simulink model "METI_Thermal_ver01_Jmaab_2018b_Intg"  (R2018b)
settings: Solver=ode8  StartTime=0  StopTime=end_time  FixedStep=sampling_time  RelTol=1e-3
PreLoadFcn:
  | %init_setting;
values from neighbouring files (symbols this model uses):
  degC2K = 273.15    [METI_TRAMI_Thermal_ver01_Jmaab_PreLoad.m]    (also in init_setting_METI.m)
  K2degC = -273.15    [METI_TRAMI_Thermal_ver01_Jmaab_PreLoad.m]    (also in init_setting_METI.m)
  sampling_time = 0.0025    [METI_TRAMI_Thermal_ver01_Jmaab_PreLoad.m]
undefined symbols (not defined in the file or in its folder): ACC_D_Gain, ACC_I_Gain, ACC_P_Gain, ALT_CNT_ALT_OFF_RPM_HYS_rpm, ALT_CNT_ALT_ON_RPM_HYS_rpm, ALT_CNT_Alter_V_BASE_V, ALT_CNT_Alter_V_Kaisei_V, ALT_CNT_flag_disable_kaisei, ALT_CNT_V_Battely_Kudo_V, ALT_PNT_ALT_GDCurrent_A, ALT_PNT_ALT_GDVolt_V, ALT_PNT_Alter_limit_Current_V_table, ALT_PNT_Alter_limit_Current_V_table_x_rpm, ALT_PNT_Alter_trq_Nm_map, ALT_PNT_Alter_trq_Nm_map_x_rpm, ALT_PNT_Alter_trq_Nm_map_y_Current_A, ALT_PNT_Alter_trq_Nm_map_z_Volt_tgt_V, ALT_PNT_eta_pulley_alt, ALT_PNT_Gain_Alt_v_del, ALT_PNT_ratio_pulley_alt, ALT_PNT_Tau_Alternator_V_tgt_s, ALT_PNT_trq_alter_output_LL_Nm, BK_PNT_Pow_UL, BK_PNT_Tau_brake, Brk_LL, Brk_PGain, Brk_UL, BT_PNT_Lo_Capa_lo_batt_F, BT_PNT_Lo_ocv_SOC_lo_batt_OCV_V_table, BT_PNT_Lo_ocv_SOC_lo_batt_OCV_V_table_x_SOC, BT_PNT_Lo_R_lo_batt_ohm, BT_PNT_Lo_SOC_MAX_lo_batt, BT_PNT_Lo_SOC_MIN_lo_batt, BT_PNT_Lo_SOC_START_lo_batt, BT_PNT_Lo_V_start_ocv, DF_PNT_DF_gear, DF_PNT_DFBlock2DFAir_Heat_Resi_KpW, DF_PNT_DFBlock_Heat_Capa_JpK, DF_PNT_DFBlock_Temp_ini_degC, DF_PNT_DFOil2DFBlock_Heat_Resi_KpW, DF_PNT_DFOil_Heat_Capa_JpK, DF_PNT_DFOil_Temp_ini_degC, DF_PNT_Driveshaft_damper, DF_PNT_Driveshaft_delta_radps_LL, DF_PNT_Driveshaft_delta_radps_UL, DF_PNT_Driveshaft_spring, DF_PNT_eta_DF, DF_PNT_Outtemp_degC, DF_PNT_TMBlock2DFBlock_Heat_Resi_KpW, Driver_Brake_Const1, Driver_Brake_Const3, Driver_Brake_Switch_Const2, Driver_Brk_sh, drivmode_ACC, drivmode_CONST, drivmode_GensokuKaisei, drivmode_GensokuRikko, drivmode_STOP, EL_PNT_R_bodyelec_lo_ohm, ENG_CNT_acc_idlestop ... (+137)
libraries: METI_Lib_vehicle_model x31, simulink x7, AZAPA_Lib_vehicle_model x1
(part 2 of 4)

== system METI_Thermal_ver01_Jmaab_2018b_Intg/Vehicle/CNT/ENG_CNT ==
  Driver_Input : Inport
  sensor_ENG_PNT : Inport  Port=2
  Bus Creator : BusCreator  Inputs=5
  Bus Creator1 : BusCreator  Inputs=10
  Bus Selector1 : BusSelector  OutputSignals=v_VL_PNT_kmph,flag_Lockup
  Bus Selector13 : BusSelector  OutputSignals=n_eng_rpm,fuel_consumption,T_ENGTH_PNT_Coolant_degC
  Bus Selector14 : BusSelector  OutputSignals=open_accel_per,open_brake_per
  ENG_Cntrl : Subsystem
  ENG_CNT_out : Outport
  tag scope: ENG_CNT_CAN_Tx=scoped
  wires:
  Bus Creator/1 -> [ENG_CNT_CAN_Tx]  "ENG_CNT_CAN_Tx"
  ENG_Cntrl/1(open_throttle_per) -> Bus Creator/1, Bus Creator1/1
  ENG_Cntrl/2(flag_IdleStop) -> Bus Creator/2, Bus Creator1/2
  ENG_Cntrl/3(flag_fuelcut) -> Bus Creator/3, Bus Creator1/3
  ENG_Cntrl/4(fuel_ratio) -> Bus Creator1/4
  ENG_Cntrl/5(timing_ignition) -> Bus Creator1/5
  ENG_Cntrl/6(n_eng_rpm) -> Bus Creator/4, Bus Creator1/6
  ENG_Cntrl/7(flag_ON_Starter) -> Bus Creator1/7
  Bus Creator1/1 -> ENG_CNT_out/1  "ENG_CNT_out"
  sensor_ENG_PNT/1 -> Bus Selector13/1
  Bus Selector13/1 -> ENG_Cntrl/3(sens_ENG_PNT)  "<n_eng_rpm>"
  Driver_Input/1 -> Bus Selector14/1
  Bus Selector14/1 -> ENG_Cntrl/1(open_accel_per)  "<open_accel_per>"
  Bus Selector14/2 -> ENG_Cntrl/2(open_brake_per)  "<open_brake_per>"
  [ENG_CNT_CAN_Rx] -> Bus Selector1/1
  Bus Selector1/2 -> ENG_Cntrl/7(flag_Lockup)  "<flag_Lockup>"
  ENG_Cntrl/8(K_Fuel) -> Bus Creator1/8
  ENG_Cntrl/9(V_ENG_CNT_WP_V) -> Bus Creator1/9
  ENG_Cntrl/10(V_ENG_CNT_RDFan_V) -> Bus Creator1/10
  Bus Selector13/2 -> ENG_Cntrl/4(fuel_consumption)  "<fuel_consumption>"
  Bus Selector13/3 -> Bus Creator/5, ENG_Cntrl/5(T_ENGTH_PNT_Coolant_degC)  "<T_ENGTH_PNT_Coolant_degC>"
  Bus Selector1/1 -> ENG_Cntrl/6(v_VL_PNT_kmph)  "<v_VL_PNT_kmph>"

== system METI_Thermal_ver01_Jmaab_2018b_Intg/Vehicle/CNT/TM_CNT ==
  sensor_TM_PNT : Inport
  Rate Transition : RateTransition  Deterministic=off
      settings: AttributesFormatString=|
      | <Integrity = %<Integrity>>
      | <Deterministic = %<Deterministic>>
  Rate Transition1 : RateTransition  Deterministic=off
      settings: AttributesFormatString=|
      | <Integrity = %<Integrity>>
      | <Deterministic = %<Deterministic>>
  Rate Transition2 : RateTransition  Deterministic=off
      settings: AttributesFormatString=|
      | <Integrity = %<Integrity>>
      | <Deterministic = %<Deterministic>>
  TM_CNT : Subsystem  TreatAsAtomicUnit=on
      settings: AttributesFormatString="<AtomicUnit =  %<TreatAsAtomicUnit>>"
  TM_CNT_out : Outport
  tag scope: TM_CNT_CAN_Tx=scoped, TM_CNT_Info=global
  wires:
  sensor_TM_PNT/1 -> Rate Transition/1
  [TM_CNT_CAN_Rx] -> Rate Transition1/1
  TM_CNT/1(TM_CNT_out) -> Rate Transition2/1
  TM_CNT/2(TM_CNT_CAN_Tx) -> [TM_CNT_CAN_Tx]
  TM_CNT/3(TM_CNT_Info) -> [TM_CNT_Info]
  Rate Transition/1 -> TM_CNT/1(sensor_TM_PNT_BUS)
  Rate Transition1/1 -> TM_CNT/2(TM_CNT_CAN_Rx)
  Rate Transition2/1 -> TM_CNT_out/1  "TM_CNT_out"

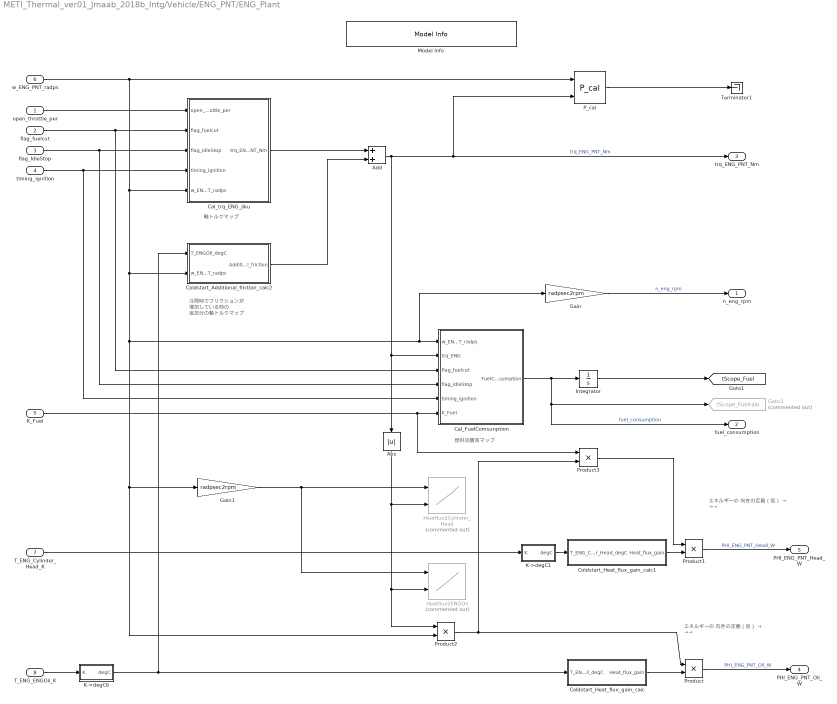
== system METI_Thermal_ver01_Jmaab_2018b_Intg/Vehicle/ENG_PNT/ENG_Plant ==
  note: 軸トルクマップ
  note: 燃料消費率マップ
  note: 冷間時でフリクションが
      | 増加している時の
      | 追加分の軸トルクマップ
  note: エネルギーの
      | 向きの定義（仮）
      | → →→
  note: エネルギーの
      | 向きの定義（仮）
      | → →→
  open_throttle_per : Inport
  flag_fuelcut : Inport  Port=2
  flag_IdleStop : Inport  Port=3
  timing_ignition : Inport  Port=4
  K_Fuel : Inport  Port=5
  w_ENG_PNT_radps : Inport  Port=6
  T_ENG_Cylinder_Head_K : Inport  Port=7
  T_ENG_ENGOil_K : Inport  Port=8
  Abs : Abs
  Add : Sum
  Cal_FuelComsunption : Subsystem
  Cal_trq_ENG_jiku : Subsystem
  Coldstart_Additional_friction_calc2 : Subsystem
  Coldstart_Heat_flux_gain_calc : Subsystem
  Coldstart_Heat_flux_gain_calc1 : Subsystem
  Gain : Gain  Gain=radpsec2rpm
  Gain1 : Gain  Gain=radpsec2rpm
  Goto3 : Goto  Commented=on  GotoTag=tScope_Fuelraio  TagVisibility=global
  Heatflux2Cylinder_Head : Lookup_n-D  Commented=on  BreakpointsForDimension1=ENG_PNT_Heatflux2Cylinder_Head_W_x_rpm  BreakpointsForDimension2=ENG_PNT_Heatflux2Cylinder_Head_W_y_trq  Table=ENG_PNT_Heatflux2Cylinder_Head_W  InternalRulePriority=Speed  RndMeth=Simplest  InputSameDT=on
  Heatflux2ENGOil : Lookup_n-D  Commented=on  BreakpointsForDimension1=ENG_PNT_Heatflux2ENGOil_W_x_rpm  BreakpointsForDimension2=ENG_PNT_Heatflux2ENGOil_W_y_trq  Table=ENG_PNT_Heatflux2ENGOil_W  InternalRulePriority=Speed  RndMeth=Simplest  InputSameDT=on
  Integrator : Integrator
  K->degC1 : Subsystem
  K->degC6 : Subsystem
  Model Info : simulink/Model-Wide Utilities/Model Info  Frame=on  DisplayStringWithTags=【注記】 ・エンジンモデルはトルク出力動作させる側が正  HorizontalTextAlignment=Left  LeftAlignmentValue=0.02
  P_cal : METI_Lib_vehicle_model/P_cal  Type_energy=回転運動  Type_output_energy=出力  Power_name=Po_  t_Workspace_Name=ENG_PNT_MECK  P_VariableName=Po_ENG_PNT_MECK  Across_VariableName=w_ENG_PNT_MECK  Throgh_VariableName=tq_ENG_PNT_MECK
  Product{,1..3} (4 alike) : Product
  Terminator1 : Terminator
  n_eng_rpm : Outport
  fuel_consumption : Outport  Port=2
  trq_ENG_PNT_Nm : Outport  Port=3
  PHI_ENG_PNT_Oil_W : Outport  Port=4
  PHI_ENG_PNT_Head_W : Outport  Port=5
  tag scope: tScope_Fuel=global
  wires:
  Cal_FuelComsunption/1(FuelConsumption) -> fuel_consumption/1, Goto3/1, Integrator/1  "fuel_consumption"
  Integrator/1 -> [tScope_Fuel]
  w_ENG_PNT_radps/1 -> P_cal/1, Coldstart_Additional_friction_calc2/2(w_ENG_PNT_radps), Gain1/1, Product2/2, Gain/1, Cal_FuelComsunption/1(w_ENG_PNT_radps), Cal_trq_ENG_jiku/5(w_ENG_PNT_radps)
  P_cal/1 -> Terminator1/1
  flag_fuelcut/1 -> Cal_trq_ENG_jiku/2(flag_fuelcut), Cal_FuelComsunption/3(flag_fuelcut)
  flag_IdleStop/1 -> Cal_FuelComsunption/4(flag_IdleStop), Cal_trq_ENG_jiku/3(flag_IdleStop)
  open_throttle_per/1 -> Cal_trq_ENG_jiku/1(open_throttle_per)
  Cal_trq_ENG_jiku/1(trq_ENG_PNT_Nm) -> Add/1
  timing_ignition/1 -> Cal_FuelComsunption/5(timing_ignition), Cal_trq_ENG_jiku/4(timing_ignition)
  Gain/1 -> n_eng_rpm/1  "n_eng_rpm"
  K->degC6/1(degC) -> Coldstart_Heat_flux_gain_calc/1(T_ENGOil_degC), Coldstart_Additional_friction_calc2/1(T_ENGOil_degC)
  T_ENG_Cylinder_Head_K/1 -> K->degC1/1(K)
  Product1/1 -> PHI_ENG_PNT_Head_W/1  "PHI_ENG_PNT_Head_W"
  Product/1 -> PHI_ENG_PNT_Oil_W/1  "PHI_ENG_PNT_Oil_W"
  Gain1/1 -> Heatflux2ENGOil/1, Heatflux2Cylinder_Head/1
  Coldstart_Heat_flux_gain_calc/1(Heat_flux_gain) -> Product/2
  Product2/1 -> Product/1, Product3/2
  Coldstart_Heat_flux_gain_calc1/1(Heat_flux_gain) -> Product1/2
  Coldstart_Additional_friction_calc2/1(Additional_friction) -> Add/2
  Add/1 -> trq_ENG_PNT_Nm/1, P_cal/2, Cal_FuelComsunption/2(trq_ENG), Abs/1  "trq_ENG_PNT_Nm"
  K_Fuel/1 -> Product3/1, Cal_FuelComsunption/6(K_Fuel)
  Abs/1 -> Product2/1, Heatflux2ENGOil/2, Heatflux2Cylinder_Head/2
  Product3/1 -> Product1/1
  T_ENG_ENGOil_K/1 -> K->degC6/1(K)
  K->degC1/1(degC) -> Coldstart_Heat_flux_gain_calc1/1(T_ENG_Cylinder_Head_degC)

== system METI_Thermal_ver01_Jmaab_2018b_Intg/Vehicle/ENG_PNT/K->degC ==
  K : Inport
  Constant2 : Constant  Value=K2degC
  Sum : Sum  Inputs=++|
  degC : Outport
  wires:
  K/1 -> Sum/2
  Constant2/1 -> Sum/1
  Sum/1 -> degC/1

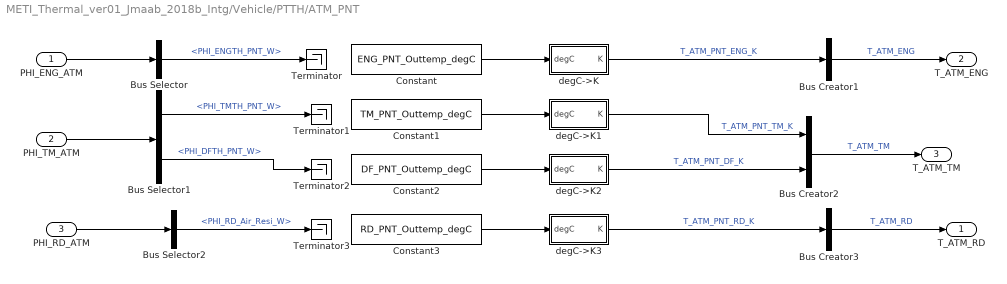
== system METI_Thermal_ver01_Jmaab_2018b_Intg/Vehicle/PTTH/ATM_PNT ==
  PHI_ENG_ATM : Inport
  PHI_TM_ATM : Inport  Port=2
  PHI_RD_ATM : Inport  Port=3
  Bus Creator1 : BusCreator  Inputs=1
  Bus Creator2 : BusCreator  Inputs=2
  Bus Creator3 : BusCreator  Inputs=1
  Bus Selector : BusSelector  OutputSignals=PHI_ENGTH_PNT_W
  Bus Selector1 : BusSelector  OutputSignals=PHI_TMTH_PNT_W,PHI_DFTH_PNT_W
  Bus Selector2 : BusSelector  OutputSignals=PHI_RD_Air_Resi_W
  Constant : Constant  Value=ENG_PNT_Outtemp_degC
  Constant1 : Constant  Value=TM_PNT_Outtemp_degC
  Constant2 : Constant  Value=DF_PNT_Outtemp_degC
  Constant3 : Constant  Value=RD_PNT_Outtemp_degC
  Terminator{,1..3} (4 alike) : Terminator
  degC->K : Subsystem
  degC->K1 : Subsystem
  degC->K2 : Subsystem
  degC->K3 : Subsystem
  T_ATM_RD : Outport
  T_ATM_ENG : Outport  Port=2
  T_ATM_TM : Outport  Port=3
  wires:
  Constant/1 -> degC->K/1(degC)
  Constant1/1 -> degC->K1/1(degC)
  Constant2/1 -> degC->K2/1(degC)
  Constant3/1 -> degC->K3/1(degC)
  Bus Selector1/2 -> Terminator2/1  "<PHI_DFTH_PNT_W>"
  degC->K/1(K) -> Bus Creator1/1  "T_ATM_PNT_ENG_K"
  degC->K1/1(K) -> Bus Creator2/1  "T_ATM_PNT_TM_K"
  degC->K2/1(K) -> Bus Creator2/2  "T_ATM_PNT_DF_K"
  degC->K3/1(K) -> Bus Creator3/1  "T_ATM_PNT_RD_K"
  PHI_ENG_ATM/1 -> Bus Selector/1
  Bus Selector/1 -> Terminator/1  "<PHI_ENGTH_PNT_W>"
  PHI_TM_ATM/1 -> Bus Selector1/1
  Bus Selector1/1 -> Terminator1/1  "<PHI_TMTH_PNT_W>"
  Bus Creator2/1 -> T_ATM_TM/1  "T_ATM_TM"
  Bus Creator1/1 -> T_ATM_ENG/1  "T_ATM_ENG"
  Bus Creator3/1 -> T_ATM_RD/1  "T_ATM_RD"
  PHI_RD_ATM/1 -> Bus Selector2/1
  Bus Selector2/1 -> Terminator3/1  "<PHI_RD_Air_Resi_W>"

== system METI_Thermal_ver01_Jmaab_2018b_Intg/Vehicle/PTTH/DTTH_PNT ==
  T_ENG_TM : Inport
  TM_CNT_out : Inport  Port=2
  PHI_TM_PNT : Inport  Port=3
  v_VL_PNT_mps : Inport  Port=4
  T_RD_TM : Inport  Port=5
  T_ATM_TM : Inport  Port=6
  DTTH_PNT : Subsystem  TreatAsAtomicUnit=on
      settings: AttributesFormatString="<AtomicUnit =  %<TreatAsAtomicUnit>>"
  Memory1 : Memory
  T_TMTH_PNT : Outport
  PHI_TM_ATM : Outport  Port=2
  PHI_TM_RD : Outport  Port=3
  PHI_TM_ENG : Outport  Port=4
  tag scope: TMTH_Info=global
  wires:
  Memory1/1 -> T_TMTH_PNT/1  "T_TMTH_PNT"
  TM_CNT_out/1 -> DTTH_PNT/1(TM_CNT_out)
  DTTH_PNT/2(PHI_TM_ENG) -> PHI_TM_ENG/1
  DTTH_PNT/1(T_TMTH_PNT) -> Memory1/1
  DTTH_PNT/5(TMTH_Info) -> [TMTH_Info]
  T_ATM_TM/1 -> DTTH_PNT/5(T_ATM_TM)
  DTTH_PNT/4(PHI_TM_ATM) -> PHI_TM_ATM/1
  PHI_TM_PNT/1 -> DTTH_PNT/2(PHI_TM_PNT)
  T_ENG_TM/1 -> DTTH_PNT/3(T_ENG_TM)
  DTTH_PNT/3(PHI_TM_RD) -> PHI_TM_RD/1
  T_RD_TM/1 -> DTTH_PNT/4(T_RD_TM)
  v_VL_PNT_mps/1 -> DTTH_PNT/6(v_VL_PNT_mps)

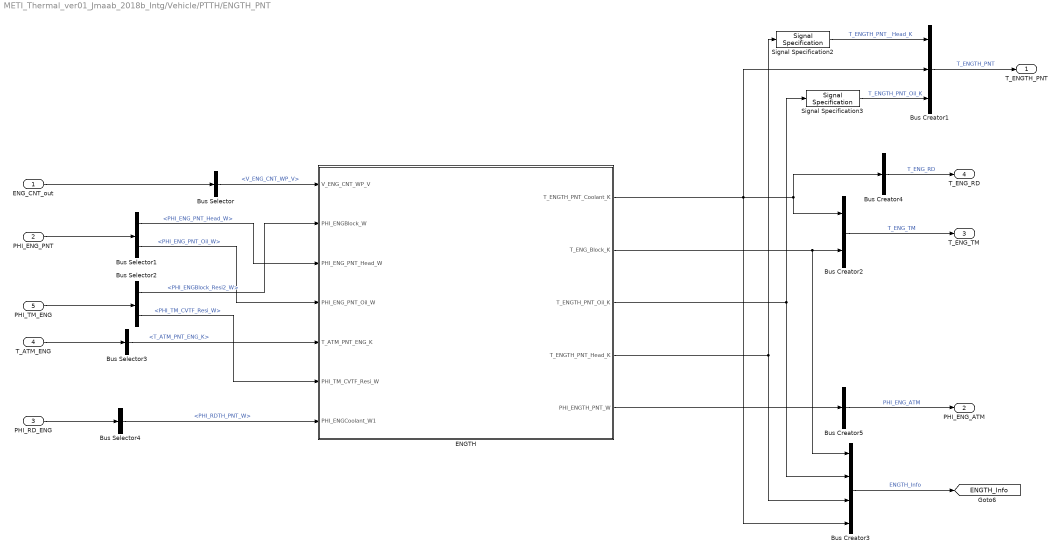
== system METI_Thermal_ver01_Jmaab_2018b_Intg/Vehicle/PTTH/ENGTH_PNT ==
  ENG_CNT_out : Inport
  PHI_ENG_PNT : Inport  Port=2
  PHI_RD_ENG : Inport  Port=3
  T_ATM_ENG : Inport  Port=4
  PHI_TM_ENG : Inport  Port=5
  Bus Creator1 : BusCreator  Inputs=3
  Bus Creator2 : BusCreator  Inputs=2
  Bus Creator3 : BusCreator  Inputs=4
  Bus Creator4 : BusCreator  Inputs=1
  Bus Creator5 : BusCreator  Inputs=1
  Bus Selector : BusSelector  OutputSignals=V_ENG_CNT_WP_V
  Bus Selector1 : BusSelector  OutputSignals=PHI_ENG_PNT_Head_W,PHI_ENG_PNT_Oil_W
  Bus Selector2 : BusSelector  OutputSignals=PHI_ENGBlock_Resi2_W,PHI_TM_CVTF_Resi_W
  Bus Selector3 : BusSelector  OutputSignals=T_ATM_PNT_ENG_K
  Bus Selector4 : BusSelector  OutputSignals=PHI_RDTH_PNT_W
  ENGTH : Subsystem
  Signal Specification2 : SignalSpecification
  Signal Specification3 : SignalSpecification
  T_ENGTH_PNT : Outport
  PHI_ENG_ATM : Outport  Port=2
  T_ENG_TM : Outport  Port=3
  T_ENG_RD : Outport  Port=4
  tag scope: ENGTH_Info=global
  wires:
  ENG_CNT_out/1 -> Bus Selector/1
  ENGTH/1(T_ENGTH_PNT_Coolant_K) -> Bus Creator3/4, Bus Creator1/2, Bus Creator2/1, Bus Creator4/1
  ENGTH/2(T_ENG_Block_K) -> Bus Creator3/1, Bus Creator2/2
  ENGTH/3(T_ENGTH_PNT_Oil_K) -> Bus Creator3/2, Signal Specification3/1
  ENGTH/4(T_ENGTH_PNT_Head_K) -> Bus Creator3/3, Signal Specification2/1
  ENGTH/5(PHI_ENGTH_PNT_W) -> Bus Creator5/1
  Bus Selector/1 -> ENGTH/1(V_ENG_CNT_WP_V)  "<V_ENG_CNT_WP_V>"
  PHI_ENG_PNT/1 -> Bus Selector1/1
  Bus Selector1/1 -> ENGTH/3(PHI_ENG_PNT_Head_W)  "<PHI_ENG_PNT_Head_W>"
  Bus Selector1/2 -> ENGTH/4(PHI_ENG_PNT_Oil_W)  "<PHI_ENG_PNT_Oil_W>"
  Bus Creator1/1 -> T_ENGTH_PNT/1  "T_ENGTH_PNT"
  Signal Specification2/1 -> Bus Creator1/1  "T_ENGTH_PNT__Head_K"
  Signal Specification3/1 -> Bus Creator1/3  "T_ENGTH_PNT_Oil_K"
  Bus Creator2/1 -> T_ENG_TM/1  "T_ENG_TM"
  Bus Creator4/1 -> T_ENG_RD/1  "T_ENG_RD"
  Bus Creator5/1 -> PHI_ENG_ATM/1  "PHI_ENG_ATM"
  Bus Creator3/1 -> [ENGTH_Info]  "ENGTH_Info"
  PHI_TM_ENG/1 -> Bus Selector2/1
  Bus Selector2/1 -> ENGTH/2(PHI_ENGBlock_W)  "<PHI_ENGBlock_Resi2_W>"
  Bus Selector2/2 -> ENGTH/6(PHI_TM_CVTF_Resi_W)  "<PHI_TM_CVTF_Resi_W>"
  T_ATM_ENG/1 -> Bus Selector3/1
  PHI_RD_ENG/1 -> Bus Selector4/1
  Bus Selector3/1 -> ENGTH/5(T_ATM_PNT_ENG_K)  "<T_ATM_PNT_ENG_K>"
  Bus Selector4/1 -> ENGTH/7(PHI_ENGCoolant_W1)  "<PHI_RDTH_PNT_W>"

== system METI_Thermal_ver01_Jmaab_2018b_Intg/Vehicle/PTTH/RDTH_PNT ==
  PHI_TM_RD : Inport
  T_ENG_RD : Inport  Port=2
  ENG_CNT_out : Inport  Port=3
  v_VL_PNT_mps : Inport  Port=4
  T_ATM_RD : Inport  Port=5
  Bus Creator : BusCreator  Inputs=1
  Bus Creator1 : BusCreator  Inputs=1
  Bus Creator2 : BusCreator  Inputs=1
  Bus Creator4 : BusCreator  Inputs=2
  Bus Selector : BusSelector  OutputSignals=V_ENG_CNT_RDFan_V
  Bus Selector1 : BusSelector  OutputSignals=T_ENGTH_PNT_Coolant_K
  Bus Selector2 : BusSelector  OutputSignals=T_ATM_PNT_RD_K
  Bus Selector3 : BusSelector  OutputSignals=PHI_Oil_TM_RD
  RDTH : Subsystem
  Terminator : Terminator
  mps2kmph : Gain  Gain=mps2kmph
  zero : Constant  Value=0
  PHI_RD_ATM : Outport
  PHI_RD_ENG : Outport  Port=2
  T_RD_TM : Outport  Port=3
  tag scope: RDTH_Info=global
  wires:
  v_VL_PNT_mps/1 -> mps2kmph/1
  RDTH/1(T_RDCoolant_degC) -> Bus Creator4/1
  RDTH/2(PHI_RDTH_PNT_W) -> Bus Creator4/2, Bus Creator1/1
  RDTH/3(PHI_RD_Air_Resi_W) -> Bus Creator2/1
  ENG_CNT_out/1 -> Bus Selector/1
  Bus Selector/1 -> RDTH/1(RD_PNT_Voltage_RDFan_V)  "<V_ENG_CNT_RDFan_V>"
  T_ENG_RD/1 -> Bus Selector1/1
  Bus Selector1/1 -> RDTH/3(T_ENGTH_PNT_Coolant_K)  "<T_ENGTH_PNT_Coolant_K>"
  mps2kmph/1 -> RDTH/2(v_VL_PNT_kmph)  "v_VL_PNT_kmph"
  Bus Creator4/1 -> [RDTH_Info]  "RDTH_Info"
  Bus Creator1/1 -> PHI_RD_ENG/1  "PHI_RD_ENG"
  Bus Creator2/1 -> PHI_RD_ATM/1  "PHI_RD_ATM"
  T_ATM_RD/1 -> Bus Selector2/1
  Bus Selector2/1 -> RDTH/4(T_ATM_PNT_RD_K)  "<T_ATM_PNT_RD_K>"
  PHI_TM_RD/1 -> Bus Selector3/1
  Bus Selector3/1 -> Terminator/1  "<PHI_Oil_TM_RD>"
  Bus Creator/1 -> T_RD_TM/1  "T_RD_TM"
  zero/1 -> Bus Creator/1  "T_PT_TH_K"

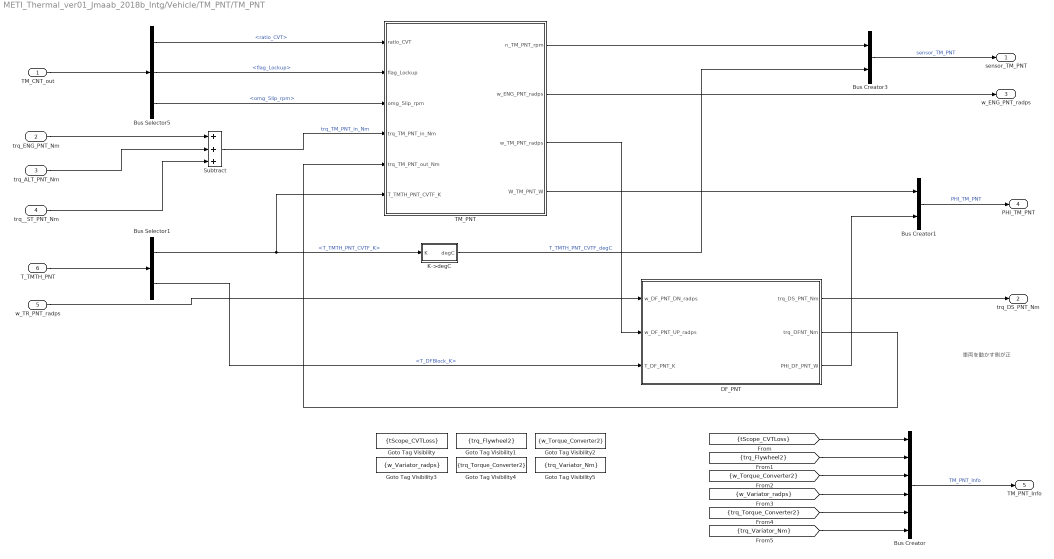
== system METI_Thermal_ver01_Jmaab_2018b_Intg/Vehicle/TM_PNT/TM_PNT ==
  note: 車両を動かす側が正
  TM_CNT_out : Inport
  trq_ENG_PNT_Nm : Inport  Port=2
  trq_ALT_PNT_Nm : Inport  Port=3
  trq__ST_PNT_Nm : Inport  Port=4
  w_TR_PNT_radps : Inport  Port=5
  T_TMTH_PNT : Inport  Port=6
  Bus Creator : BusCreator  Inputs=6
  Bus Creator1 : BusCreator  Inputs=2
  Bus Creator3 : BusCreator  Inputs=2
  Bus Selector1 : BusSelector  OutputSignals=T_TMTH_PNT_CVTF_K,T_DFBlock_K
  Bus Selector5 : BusSelector  OutputSignals=ratio_CVT,flag_Lockup,omg_Slip_rpm
  DF_PNT : Subsystem
  Goto Tag Visibility : GotoTagVisibility  GotoTag=tScope_CVTLoss
  Goto Tag Visibility1 : GotoTagVisibility  GotoTag=trq_Flywheel2
  Goto Tag Visibility2 : GotoTagVisibility  GotoTag=w_Torque_Converter2
  Goto Tag Visibility3 : GotoTagVisibility  GotoTag=w_Variator_radps
  Goto Tag Visibility4 : GotoTagVisibility  GotoTag=trq_Torque_Converter2
  Goto Tag Visibility5 : GotoTagVisibility  GotoTag=trq_Variator_Nm
  K->degC : Subsystem
  Subtract : Sum  Inputs=3
  TM_PNT : Subsystem
  sensor_TM_PNT : Outport
  trq_DS_PNT_Nm : Outport  Port=2
  w_ENG_PNT_radps : Outport  Port=3
  PHI_TM_PNT : Outport  Port=4
  TM_PNT_Info : Outport  Port=5
  wires:
  DF_PNT/3(PHI_DF_PNT_W) -> Bus Creator1/2
  TM_PNT/4(W_TM_PNT_W) -> Bus Creator1/1
  Bus Selector5/3 -> TM_PNT/3(omg_Slip_rpm)  "<omg_Slip_rpm>"
  trq_ENG_PNT_Nm/1 -> Subtract/1
  Bus Creator3/1 -> sensor_TM_PNT/1  "sensor_TM_PNT"
  trq__ST_PNT_Nm/1 -> Subtract/3
  TM_PNT/2(w_ENG_PNT_radps) -> w_ENG_PNT_radps/1
  K->degC/1(degC) -> Bus Creator3/2  "T_TMTH_PNT_CVTF_degC"
  Bus Selector5/2 -> TM_PNT/2(flag_Lockup)  "<flag_Lockup>"
  Bus Selector1/1 -> TM_PNT/6(T_TMTH_PNT_CVTF_K), K->degC/1(K)  "<T_TMTH_PNT_CVTF_K>"
  DF_PNT/2(trq_DFNT_Nm) -> TM_PNT/5(trq_TM_PNT_out_Nm)
  Bus Selector5/1 -> TM_PNT/1(ratio_CVT)  "<ratio_CVT>"
  trq_ALT_PNT_Nm/1 -> Subtract/2
  TM_PNT/1(n_TM_PNT_rpm) -> Bus Creator3/1
  T_TMTH_PNT/1 -> Bus Selector1/1
  DF_PNT/1(trq_DS_PNT_Nm) -> trq_DS_PNT_Nm/1
  TM_PNT/3(w_TM_PNT_radps) -> DF_PNT/2(w_DF_PNT_UP_radps)
  Bus Creator1/1 -> PHI_TM_PNT/1  "PHI_TM_PNT"
  w_TR_PNT_radps/1 -> DF_PNT/1(w_DF_PNT_DN_radps)
  Subtract/1 -> TM_PNT/4(trq_TM_PNT_in_Nm)  "trq_TM_PNT_in_Nm"
  Bus Selector1/2 -> DF_PNT/3(T_DF_PNT_K)  "<T_DFBlock_K>"
  TM_CNT_out/1 -> Bus Selector5/1
  Bus Creator/1 -> TM_PNT_Info/1  "TM_PNT_Info"
  [tScope_CVTLoss] -> Bus Creator/1
  [trq_Flywheel2] -> Bus Creator/2
  [w_Torque_Converter2] -> Bus Creator/3
  [w_Variator_radps] -> Bus Creator/4
  [trq_Torque_Converter2] -> Bus Creator/5
  [trq_Variator_Nm] -> Bus Creator/6

== system METI_Thermal_ver01_Jmaab_2018b_Intg/Driver/Caliculate_Opeining_Accel/FB/Filter ==
  In1 : Inport
  Gain3 : Gain  Gain=10
  Gain4 : Gain  Gain=0.1
  Rounding Function : Rounding  Operator=round
  Out1 : Outport
  wires:
  Rounding Function/1 -> Gain4/1
  In1/1 -> Gain3/1
  Gain3/1 -> Rounding Function/1
  Gain4/1 -> Out1/1

== system METI_Thermal_ver01_Jmaab_2018b_Intg/Driver/Caliculate_Opeining_Accel/FF/Air_Resistance ==
  V_tgt : Inport
  V_wind : Constant  Value=VL_PNT_V_wind
  cal_Air_resi1 : METI_Lib_vehicle_model/vehicle_model/cal_Air_resi  Vel_max=200
  F_air_resi : Outport
  wires:
  V_tgt/1 -> cal_Air_resi1/1
  V_wind/1 -> cal_Air_resi1/2
  cal_Air_resi1/1 -> F_air_resi/1

== system METI_Thermal_ver01_Jmaab_2018b_Intg/Driver/Caliculate_Opeining_Accel/FF/Cal_M_ENG_jiku2 ==
  note: 軸トルクマップ
  FF_trq_accel_Nm : Inport
  pre_n_eng_rpm : Inport  Port=2
  2-D Lookup Table : Lookup_n-D  BreakpointsForDimension1=ENG_trq_rev  BreakpointsForDimension2=ENG_rpm  Table=ENG_throttle_rev  ExtrapMethod=Clip  UseLastTableValue=on  RndMeth=Simplest  InputSameDT=on
  2-D Lookup Table1 : Lookup_n-D  BreakpointsForDimension1=ENG_PNT_trq_Nm_map_y_throttle  BreakpointsForDimension2=ENG_PNT_trq_Nm_map_x_rpm  Table=ENG_PNT_trq_Nm_map  ExtrapMethod=Clip  UseLastTableValue=on  RndMeth=Simplest  InputSameDT=on
  Constant : Constant  Value=0
  Subsystem : Subsystem
  Sum : Sum  Inputs=|++
  FF_open_accel_per : Outport
  wires:
  FF_trq_accel_Nm/1 -> Sum/1
  2-D Lookup Table/1 -> Subsystem/1(In1)
  pre_n_eng_rpm/1 -> 2-D Lookup Table/2, 2-D Lookup Table1/2
  Constant/1 -> 2-D Lookup Table1/1
  Sum/1 -> 2-D Lookup Table/1
  2-D Lookup Table1/1 -> Sum/2
  Subsystem/1(Out1) -> FF_open_accel_per/1

== system METI_Thermal_ver01_Jmaab_2018b_Intg/Driver/Caliculate_Opeining_Accel/FF/Inertial_Resistance ==
  V_tgt : Inport
  Constant : Constant  Value=M
  Derivative : Derivative
  Divide : Product  OutDataTypeStr=Inherit: Same as first input
  F_Inertia : Outport
  wires:
  Constant/1 -> Divide/2
  Derivative/1 -> Divide/1
  Divide/1 -> F_Inertia/1
  V_tgt/1 -> Derivative/1

== system METI_Thermal_ver01_Jmaab_2018b_Intg/Driver/Caliculate_Opeining_Accel/FF/Rolling_Resistance ==
  note: 20151211修正
      |
      | 空気抵抗と表現を統一する、ため
      | -1のGainを削除
  V_tgt : Inport
  cal_roll_resi1 : METI_Lib_vehicle_model/vehicle_model/cal_roll_resi  Myu_tire=myu  Vehicle_Mass=M  Gravi_acc=g
  F_rollresi : Outport
  wires:
  V_tgt/1 -> cal_roll_resi1/1
  cal_roll_resi1/1 -> F_rollresi/1

== system METI_Thermal_ver01_Jmaab_2018b_Intg/Vehicle/ALT_PNT/Subsystem/I_alt_cal ==
  target_volt_ALT_V : Inport
  volt_BT_PNT_Lo_V : Inport  Port=2
  rpm_alt : Inport  Port=3
  Add : Sum
  Cal_I_alt_P_control : Subsystem
  Cal_I_alt_base : Subsystem
  Constant : Constant  Value=12
  Constant4 : Constant  Value=0
  Limit_Current_Max : Lookup_n-D  NumberOfTableDimensions=1  BreakpointsForDimension1=ALT_PNT_Alter_limit_Current_V_table_x_rpm  Table=ALT_PNT_Alter_limit_Current_V_table  ExtrapMethod=Clip  UseLastTableValue=on  RndMeth=Simplest  InputSameDT=on
  MinMax2 : MinMax  Function=max  Inputs=2
  Sum1 : Sum  Inputs=|+-
  Sum2 : Sum  Inputs=-+|
  電圧比較 : MinMax  Inputs=2
  I_alt : Outport
  wires:
  target_volt_ALT_V/1 -> Sum1/1, Sum2/2
  volt_BT_PNT_Lo_V/1 -> Sum2/1
  rpm_alt/1 -> Limit_Current_Max/1
  Constant4/1 -> MinMax2/2
  Limit_Current_Max/1 -> MinMax2/1  "I_limit_ALT"
  電圧比較/1 -> I_alt/1
  Add/1 -> 電圧比較/2
  Sum2/1 -> Cal_I_alt_P_control/1(V_delt_tgt)
  MinMax2/1 -> 電圧比較/1
  Constant/1 -> Sum1/2
  Sum1/1 -> Cal_I_alt_base/1(V_delt_tgt)
  Cal_I_alt_P_control/1(I_alt_base) -> Add/1
  Cal_I_alt_base/1(I_alt_base) -> Add/2

== system METI_Thermal_ver01_Jmaab_2018b_Intg/Vehicle/ALT_PNT/Subsystem/Torque_Guard ==
  current_ALT_PNT_A : Inport
  V_ALT_PNT : Inport  Port=2
  n_ROT_slavepulley12_rpm : Inport  Port=3
  ALT_GDCurrent : Inport  Port=4
  ALT_GDVolt : Inport  Port=5
  Caliculate_Axes_Torque1 : Lookup_n-D  NumberOfTableDimensions=3  BreakpointsForDimension1=ALT_PNT_Alter_trq_Nm_map_x_rpm  BreakpointsForDimension2=ALT_PNT_Alter_trq_Nm_map_y_Current_A  BreakpointsForDimension3=ALT_PNT_Alter_trq_Nm_map_z_Volt_tgt_V  Table=ALT_PNT_Alter_trq_Nm_map  RndMeth=Simplest  InputSameDT=on
  Caliculate_Axes_Torque2 : Lookup_n-D  NumberOfTableDimensions=3  BreakpointsForDimension1=ALT_PNT_Alter_trq_Nm_map_x_rpm  BreakpointsForDimension2=ALT_PNT_Alter_trq_Nm_map_y_Current_A  BreakpointsForDimension3=ALT_PNT_Alter_trq_Nm_map_z_Volt_tgt_V  Table=ALT_PNT_Alter_trq_Nm_map  RndMeth=Simplest  InputSameDT=on
  Constant3 : Constant  Value=ALT_PNT_trq_alter_output_LL_Nm
  MinMax : MinMax  Inputs=2
  MinMax1 : MinMax  Function=max  Inputs=2
  trq_trqsource : Outport
  wires:
  ALT_GDCurrent/1 -> Caliculate_Axes_Torque2/2
  Caliculate_Axes_Torque2/1 -> MinMax/2
  MinMax/1 -> MinMax1/1
  Caliculate_Axes_Torque1/1 -> MinMax/1
  Constant3/1 -> MinMax1/2
  ALT_GDVolt/1 -> Caliculate_Axes_Torque2/3
  MinMax1/1 -> trq_trqsource/1
  V_ALT_PNT/1 -> Caliculate_Axes_Torque1/3
  current_ALT_PNT_A/1 -> Caliculate_Axes_Torque1/2
  n_ROT_slavepulley12_rpm/1 -> Caliculate_Axes_Torque2/1, Caliculate_Axes_Torque1/1

== system METI_Thermal_ver01_Jmaab_2018b_Intg/Vehicle/BT_PNT_Lo/Cal_SOC/Subsystem4 ==
  In1 : Inport
  In2 : Inport  Port=2
  To Workspace : ToWorkspace  VariableName=SOC_LoBat  SampleTime=-1
      settings: Decimation=num_tws_mabiki
  To Workspace1 : ToWorkspace  VariableName=Asec_LoBat  SampleTime=-1
      settings: Decimation=num_tws_mabiki
  wires:
  In1/1 -> To Workspace/1
  In2/1 -> To Workspace1/1

== system METI_Thermal_ver01_Jmaab_2018b_Intg/Vehicle/CNT/ALT_CNT/ALT_Ctrl ==
  note: 【発電禁止条件】
      | 下記条件いずれかが成立時はオルタネータの発電を禁止する
      |   (2)エンジン停止中
      |   (3)エンジン始動中(下記エンジン回転数で判定)
      |      ene ≦ ALT_ON_RPM_HYS(1000[rpm])
      |                    ヒスあり(400[rpm])
  note: 【強制回生モード切替条件】
  note: 【回生モード切替条件】
      | 減速時FC中
  note: 例) 12[V]
  note: 例) 14[V]
  note: 例) 13.5[V]
  SOC_BT_PNT_Lo_PCT : Inport
  flag_fuelcut : Inport  Port=2
  flag_IdleStop : Inport  Port=3
  n_eng_rpm : Inport  Port=4
  Constant : Constant  Value=ALT_CNT_Alter_V_Kaisei_V
  Constant1 : Constant  Value=ALT_CNT_V_Battely_Kudo_V
  Constant2 : Constant  Value=ALT_CNT_flag_disable_kaisei
  Constant3 : Constant  Value=ALT_CNT_Alter_V_BASE_V
  Constant4 : Constant  Value=BT_PNT_Lo_SOC_MAX_lo_batt
  Logical Operator : Logic  Operator=OR  Inputs=3  AllPortsSameDT=off  OutDataTypeStr=boolean
  Logical Operator1 : Logic  AllPortsSameDT=off  OutDataTypeStr=boolean
  Logical Operator2 : Logic  Operator=NOT  AllPortsSameDT=off  OutDataTypeStr=boolean
  Relational Operator : RelationalOperator  OutDataTypeStr=boolean  RndMeth=Nearest
  Relay1 : Relay  OnSwitchValue=ALT_CNT_ALT_ON_RPM_HYS_rpm  OffSwitchValue=ALT_CNT_ALT_OFF_RPM_HYS_rpm  OnOutputValue=0  OffOutputValue=1
  Switch1 : Switch  Criteria=u2 > Threshold  Threshold=0.5
  Switch3 : Switch  Criteria=u2 > Threshold  Threshold=0.5
  target_volt_ALT_V : Outport
  wires:
  Switch3/1 -> target_volt_ALT_V/1  "target_volt_ALT_V"
  Constant3/1 -> Switch3/1
  Logical Operator2/1 -> Logical Operator1/2
  SOC_BT_PNT_Lo_PCT/1 -> Relational Operator/1
  Constant2/1 -> Switch3/2
  flag_fuelcut/1 -> Logical Operator1/1
  Relational Operator/1 -> Logical Operator/3
  Constant4/1 -> Relational Operator/2
  Logical Operator1/1 -> Switch1/2
  Logical Operator/1 -> Logical Operator2/1
  Constant/1 -> Switch1/1
  Relay1/1 -> Logical Operator/2
  Switch1/1 -> Switch3/3
  Constant1/1 -> Switch1/3
  flag_IdleStop/1 -> Logical Operator/1
  n_eng_rpm/1 -> Relay1/1

== system METI_Thermal_ver01_Jmaab_2018b_Intg/Vehicle/CNT/BK_CNT/BK_Ctrl ==
  open_brake_per_in : Inport
  v_VL_PNT_kmph_in : Inport  Port=2
  trq_BK_PNT_Nm_in : Inport  Port=3
  open_brake_per : Outport
  v_VL_PNT_kmph : Outport  Port=2
  trq_BK_PNT_Nm : Outport  Port=3
  wires:
  v_VL_PNT_kmph_in/1 -> v_VL_PNT_kmph/1
  trq_BK_PNT_Nm_in/1 -> trq_BK_PNT_Nm/1
  open_brake_per_in/1 -> open_brake_per/1

== system METI_Thermal_ver01_Jmaab_2018b_Intg/Vehicle/CNT/CAN/ALT_CNT ==
  note: ALT_Ctrl
  Pwtr_CAN : Inport
  Bus Creator2 : BusCreator  Inputs=3
  Bus Selector3 : BusSelector  OutputSignals=ENG_CNT_CAN_Tx
  Bus Selector4 : BusSelector  OutputSignals=flag_fuelcut,flag_IdleStop,n_eng_rpm
  tag scope: ALT_CNT_CAN_Rx=scoped
  wires:
  Bus Selector4/2 -> Bus Creator2/2  "<flag_IdleStop>"
  Bus Selector4/3 -> Bus Creator2/3  "<n_eng_rpm>"
  Pwtr_CAN/1 -> Bus Selector3/1
  Bus Creator2/1 -> [ALT_CNT_CAN_Rx]  "ALT_CNT_CAN_Rx"
  Bus Selector4/1 -> Bus Creator2/1  "<flag_fuelcut>"
  Bus Selector3/1 -> Bus Selector4/1  "<ENG_CNT_CAN_Tx>"

== system METI_Thermal_ver01_Jmaab_2018b_Intg/Vehicle/CNT/CAN/BK_CNT ==
  note: BK_Ctrl
  Pwtr_CAN : Inport
  Terminator : Terminator
  BK_CNT_CAN_Tx : Outport
  wires:
  [BK_CNT_CAN_Tx] -> BK_CNT_CAN_Tx/1
  Pwtr_CAN/1 -> Terminator/1

== system METI_Thermal_ver01_Jmaab_2018b_Intg/Vehicle/CNT/CAN/ENG_CNT ==
  note: ENG_Ctrl
  Pwtr_CAN : Inport
  Bus Creator3 : BusCreator  Inputs=2
  Bus Selector1 : BusSelector  OutputSignals=TM_CNT_CAN_Tx,BK_CNT_CAN_Tx
  Bus Selector2 : BusSelector  OutputSignals=flag_Lockup
  Bus Selector3 : BusSelector  OutputSignals=v_VL_PNT_kmph
  ENG_CNT_CAN_Tx : Outport
  tag scope: ENG_CNT_CAN_Rx=scoped
  wires:
  Bus Creator3/1 -> [ENG_CNT_CAN_Rx]  "ENG_CNT_CAN_Rx"
  Bus Selector1/1 -> Bus Selector2/1  "<TM_CNT_CAN_Tx>"
  Bus Selector2/1 -> Bus Creator3/1  "<flag_Lockup>"
  Pwtr_CAN/1 -> Bus Selector1/1
  [ENG_CNT_CAN_Tx] -> ENG_CNT_CAN_Tx/1
  Bus Selector1/2 -> Bus Selector3/1  "<BK_CNT_CAN_Tx>"
  Bus Selector3/1 -> Bus Creator3/2  "<v_VL_PNT_kmph>"

== system METI_Thermal_ver01_Jmaab_2018b_Intg/Vehicle/CNT/CAN/Pwtr_CAN ==
  note: 通信遅れ無し
  ENG_CNT_CAN_Tx : Inport
  TM_CNT_CAN_Tx : Inport  Port=2
  BK_CNT_CAN_Tx : Inport  Port=3
  Bus Creator8 : BusCreator  Inputs=3
  Unit Delay : UnitDelay  SampleTime=-1
  Pwtr_CAN : Outport
  wires:
  ENG_CNT_CAN_Tx/1 -> Bus Creator8/1
  TM_CNT_CAN_Tx/1 -> Bus Creator8/2
  Unit Delay/1 -> Pwtr_CAN/1  "Pwtr_CAN"
  Bus Creator8/1 -> Unit Delay/1
  BK_CNT_CAN_Tx/1 -> Bus Creator8/3

== system METI_Thermal_ver01_Jmaab_2018b_Intg/Vehicle/CNT/CAN/TM_CNT ==
  note: TM_Ctrl
  Pwtr_CAN : Inport
  Bus Creator4 : BusCreator  Inputs=3
  Bus Selector3 : BusSelector  OutputSignals=v_VL_PNT_kmph
  Bus Selector5 : BusSelector  OutputSignals=ENG_CNT_CAN_Tx,BK_CNT_CAN_Tx
  Bus Selector6 : BusSelector  OutputSignals=open_throttle_per,T_ENGTH_PNT_Coolant_degC
  TM_CNT_CAN_Tx : Outport
  tag scope: TM_CNT_CAN_Rx=scoped
  wires:
  Bus Selector5/1 -> Bus Selector6/1  "<ENG_CNT_CAN_Tx>"
  Bus Selector6/1 -> Bus Creator4/1  "<open_throttle_per>"
  Pwtr_CAN/1 -> Bus Selector5/1
  Bus Creator4/1 -> [TM_CNT_CAN_Rx]  "TM_CNT_CAN_Rx"
  [TM_CNT_CAN_Tx] -> TM_CNT_CAN_Tx/1
  Bus Selector6/2 -> Bus Creator4/2  "<T_ENGTH_PNT_Coolant_degC>"
  Bus Selector5/2 -> Bus Selector3/1  "<BK_CNT_CAN_Tx>"
  Bus Selector3/1 -> Bus Creator4/3  "<v_VL_PNT_kmph>"

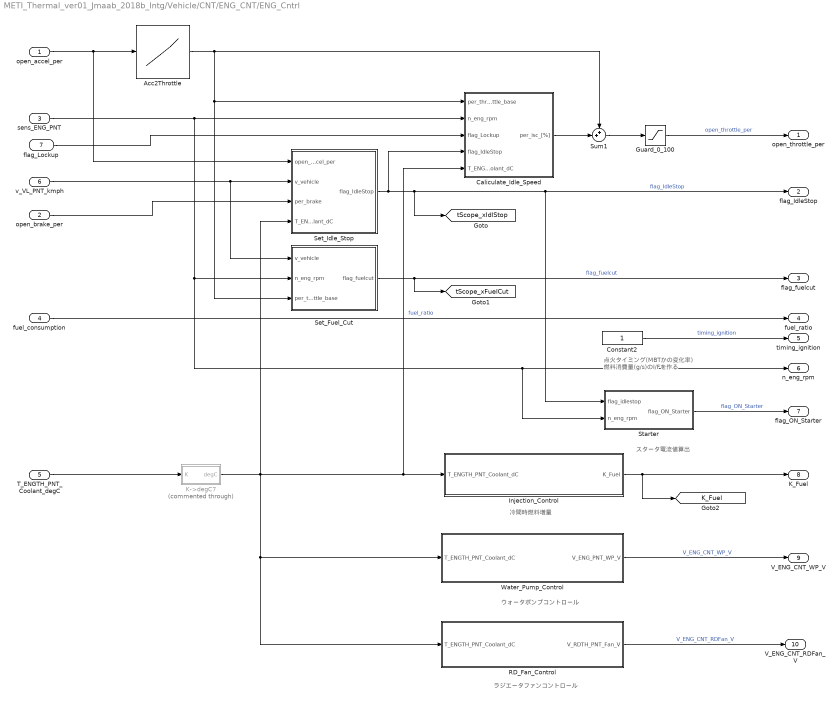
== system METI_Thermal_ver01_Jmaab_2018b_Intg/Vehicle/CNT/ENG_CNT/ENG_Cntrl ==
  note: 点火タイミング(MBTかの変化率)
      | 燃料消費量(g/s)のI/Fを作る
  note: スタータ電流値算出
  note: 冷間時燃料増量
  note: ウォータポンプコントロール
  note: ラジエータファンコントロール
  open_accel_per : Inport
  open_brake_per : Inport  Port=2
  sens_ENG_PNT : Inport  Port=3
  fuel_consumption : Inport  Port=4
  T_ENGTH_PNT_Coolant_degC : Inport  Port=5
  v_VL_PNT_kmph : Inport  Port=6
  flag_Lockup : Inport  Port=7
  Acc2Throttle : Lookup_n-D  NumberOfTableDimensions=1  BreakpointsForDimension1=[ENG_CNT_Accel_LL:ENG_CNT_Accel_UL]  Table=[ENG_CNT_Throttle_LL:ENG_CNT_Throttle_UL]  RndMeth=Simplest  InputSameDT=on
  Caliculate_Idle_Speed : Subsystem
  Constant2 : Constant
  Guard_0_100 : Saturate  UpperLimit=ENG_CNT_Throttle_UL  LowerLimit=ENG_CNT_Throttle_LL
  Injection_Control : Subsystem
  K->degC7 : Subsystem  Commented=through
  RD_Fan_Control : Subsystem
  Set_Fuel_Cut : Subsystem
  Set_Idle_Stop : Subsystem
  Starter : Subsystem
  Sum1 : Sum  Inputs=++|
  Water_Pump_Control : Subsystem
  open_throttle_per : Outport
  flag_IdleStop : Outport  Port=2
  flag_fuelcut : Outport  Port=3
  fuel_ratio : Outport  Port=4
  timing_ignition : Outport  Port=5
  n_eng_rpm : Outport  Port=6
  flag_ON_Starter : Outport  Port=7
  K_Fuel : Outport  Port=8
  V_ENG_CNT_WP_V : Outport  Port=9
  V_ENG_CNT_RDFan_V : Outport  Port=10
  tag scope: K_Fuel=global, tScope_xFuelCut=global, tScope_xIdlStop=global
  wires:
  Set_Idle_Stop/1(flag_IdleStop) -> [tScope_xIdlStop], Starter/1(flag_idlestop), flag_IdleStop/1, Caliculate_Idle_Speed/4(flag_IdleStop)  "flag_IdleStop"
  Caliculate_Idle_Speed/1(per_isc_[%]) -> Sum1/2
  Sum1/1 -> Guard_0_100/1
  Acc2Throttle/1 -> Sum1/1, Caliculate_Idle_Speed/1(per_throttle_base), Set_Fuel_Cut/3(per_throttle_base)
  fuel_consumption/1 -> fuel_ratio/1  "fuel_ratio"
  Constant2/1 -> timing_ignition/1  "timing_ignition"
  Set_Fuel_Cut/1(flag_fuelcut) -> flag_fuelcut/1, [tScope_xFuelCut]  "flag_fuelcut"
  Guard_0_100/1 -> open_throttle_per/1  "open_throttle_per"
  sens_ENG_PNT/1 -> Caliculate_Idle_Speed/2(n_eng_rpm), Set_Fuel_Cut/2(n_eng_rpm), n_eng_rpm/1, Starter/2(n_eng_rpm)
  open_brake_per/1 -> Set_Idle_Stop/3(per_brake)
  open_accel_per/1 -> Acc2Throttle/1, Set_Idle_Stop/1(open_accel_per)
  v_VL_PNT_kmph/1 -> Set_Fuel_Cut/1(v_vehicle), Set_Idle_Stop/2(v_vehicle)
  Starter/1(flag_ON_Starter) -> flag_ON_Starter/1  "flag_ON_Starter"
  flag_Lockup/1 -> Caliculate_Idle_Speed/3(flag_Lockup)
  Water_Pump_Control/1(V_ENG_PNT_WP_V) -> V_ENG_CNT_WP_V/1  "V_ENG_CNT_WP_V"
  T_ENGTH_PNT_Coolant_degC/1 -> K->degC7/1(K)
  Injection_Control/1(K_Fuel) -> [K_Fuel], K_Fuel/1
  RD_Fan_Control/1(V_RDTH_PNT_Fan_V) -> V_ENG_CNT_RDFan_V/1  "V_ENG_CNT_RDFan_V"
  K->degC7/1(degC) -> RD_Fan_Control/1(T_ENGTH_PNT_Coolant_dC), Water_Pump_Control/1(T_ENGTH_PNT_Coolant_dC), Set_Idle_Stop/4(T_ENGTH_PNT_Coolant_dC), Injection_Control/1(T_ENGTH_PNT_Coolant_dC), Caliculate_Idle_Speed/5(T_ENGTH_PNT_Coolant_dC)

== system METI_Thermal_ver01_Jmaab_2018b_Intg/Vehicle/CNT/TM_CNT/TM_CNT ==
  sensor_TM_PNT_BUS : Inport  SampleTime=0.01
      settings: AttributesFormatString=<SampleTime = %<SampleTime>>
  TM_CNT_CAN_Rx : Inport  Port=2  SampleTime=0.01
      settings: AttributesFormatString=<SampleTime = %<SampleTime>>
  Bus Creator : BusCreator  Inputs=2
  Bus Creator1 : BusCreator  Inputs=4
  Bus Creator2 : BusCreator  Inputs=2
  Bus Selector1 : BusSelector  OutputSignals=v_VL_PNT_kmph,T_ENGTH_PNT_Coolant_degC,open_throttle_per
  Bus Selector2 : BusSelector  OutputSignals=n_TM_PNT_rpm,T_TMTH_PNT_CVTF_degC
  Goto Tag Visibility : GotoTagVisibility  GotoTag=tScope_Luckup
  Goto Tag Visibility1 : GotoTagVisibility  GotoTag=tScope_CVTratio
  TM_Ctrl : Subsystem
  TM_CNT_out : Outport
  TM_CNT_CAN_Tx : Outport  Port=2
  TM_CNT_Info : Outport  Port=3
  wires:
  Bus Selector2/2 -> TM_Ctrl/3(T_TMTH_PNT_CVTF_degC)  "<T_TMTH_PNT_CVTF_degC>"
  Bus Selector1/3 -> TM_Ctrl/5(open_throttle_per)  "<open_throttle_per>"
  TM_Ctrl/2(omg_Slip_rpm) -> Bus Creator1/2, Bus Creator/2
  Bus Selector1/1 -> TM_Ctrl/1(v_VL_PNT_kmph)  "<v_VL_PNT_kmph>"
  [tScope_Luckup] -> Bus Creator2/1
  TM_Ctrl/1(flag_Lockup) -> Bus Creator1/1, Bus Creator/1
  [tScope_CVTratio] -> Bus Creator2/2
  Bus Selector2/1 -> TM_Ctrl/2(n_TM_PNT_rpm)  "<n_TM_PNT_rpm>"
  TM_Ctrl/3(ratio_CVT) -> Bus Creator1/3
  Bus Creator1/1 -> TM_CNT_out/1  "TM_CNT_out"
  sensor_TM_PNT_BUS/1 -> Bus Selector2/1
  TM_Ctrl/4(R_CVTF_warmer_tgt_KpW) -> Bus Creator1/4
  Bus Selector1/2 -> TM_Ctrl/4(T_ENGTH_PNT_Coolant_degC)  "<T_ENGTH_PNT_Coolant_degC>"
  Bus Creator2/1 -> TM_CNT_Info/1  "TM_CNT_Info"
  TM_CNT_CAN_Rx/1 -> Bus Selector1/1
  Bus Creator/1 -> TM_CNT_CAN_Tx/1  "TM_CNT_CAN_Tx"

== system METI_Thermal_ver01_Jmaab_2018b_Intg/Vehicle/ENG_PNT/ENG_Plant/Cal_FuelComsunption ==
  w_ENG_PNT_radps : Inport
  trq_ENG : Inport  Port=2
  flag_fuelcut : Inport  Port=3
  flag_IdleStop : Inport  Port=4
  timing_ignition : Inport  Port=5
  K_Fuel : Inport  Port=6
  1-D Lookup Table1 : Lookup_n-D  NumberOfTableDimensions=1  BreakpointsForDimension1=ENG_PNT_trq_fluc_Nm_table_x_spk_tim  Table=ENG_PNT_trq_fluc_Nm_table  RndMeth=Simplest  InputSameDT=on
  Map_FuelRate : Lookup_n-D  BreakpointsForDimension1=ENG_PNT_FuelCon_gps_map_y_trq_Nm  BreakpointsForDimension2=ENG_PNT_FuelCon_gps_map_x_pri_rpm  Table=ENG_PNT_FuelCon_gps_map  RndMeth=Simplest  InputSameDT=on
  Not_cal1 : Subsystem
  Not_cal2 : Subsystem
  Product : Product  Inputs=4  RndMeth=Zero
  Product1 : Product  Inputs=*/  RndMeth=Zero
  radpsec2rpm : Gain  Gain=radpsec2rpm
  FuelConsumption : Outport
  wires:
  trq_ENG/1 -> Product1/1
  radpsec2rpm/1 -> Map_FuelRate/2
  w_ENG_PNT_radps/1 -> radpsec2rpm/1
  Product/1 -> FuelConsumption/1
  Not_cal2/1(Out1) -> Product/3
  Not_cal1/1(Out1) -> Product/2
  flag_fuelcut/1 -> Not_cal1/1(In1)
  flag_IdleStop/1 -> Not_cal2/1(In1)
  timing_ignition/1 -> 1-D Lookup Table1/1
  1-D Lookup Table1/1 -> Product1/2
  Product1/1 -> Map_FuelRate/1
  Map_FuelRate/1 -> Product/1
  K_Fuel/1 -> Product/4

== system METI_Thermal_ver01_Jmaab_2018b_Intg/Vehicle/ENG_PNT/ENG_Plant/Cal_trq_ENG_jiku ==
  note: エンジン軸トルクマップ
  open_throttle_per : Inport
  flag_fuelcut : Inport  Port=2
  flag_IdleStop : Inport  Port=3
  timing_ignition : Inport  Port=4
  w_ENG_PNT_radps : Inport  Port=5
  1-D Lookup Table : Lookup_n-D  NumberOfTableDimensions=1  BreakpointsForDimension1=ENG_PNT_trq_fluc_Nm_table_x_spk_tim  Table=ENG_PNT_trq_fluc_Nm_table  RndMeth=Simplest  InputSameDT=on
  2-D Lookup Table : Lookup_n-D  BreakpointsForDimension1=ENG_PNT_trq_Nm_map_y_throttle  BreakpointsForDimension2=ENG_PNT_trq_Nm_map_x_rpm  Table=ENG_PNT_trq_Nm_map  ExtrapMethod=Clip  UseLastTableValue=on  RndMeth=Simplest  InputSameDT=on
  Model Info : simulink/Model-Wide Utilities/Model Info  Frame=on  DisplayStringWithTags=|  HorizontalTextAlignment=Left  LeftAlignmentValue=0.02
      | 【注記】
      | ・燃料カット時はスロットル開度を0としてエンジンフリクションを付加
      | ・点火タイミングによるトルク変動を想定
      | ・エンジン軸トルクマップの使用
  Not_cal : Subsystem
  Not_cal1 : Subsystem
  Product : Product  RndMeth=Zero
  Product1 : Product  RndMeth=Zero
  Product2 : Product  RndMeth=Zero
  Saturation : Saturate  UpperLimit=ENG_CNT_Throttle_UL  LowerLimit=ENG_CNT_Throttle_LL
  radpsec2rpm : Gain  Gain=radpsec2rpm
  trq_ENG_PNT_Nm : Outport
  wires:
  w_ENG_PNT_radps/1 -> radpsec2rpm/1
  2-D Lookup Table/1 -> Product1/1
  open_throttle_per/1 -> Product/1
  Saturation/1 -> 2-D Lookup Table/1
  radpsec2rpm/1 -> 2-D Lookup Table/2
  timing_ignition/1 -> 1-D Lookup Table/1
  1-D Lookup Table/1 -> Product1/2
  Product/1 -> Saturation/1
  Product2/1 -> Product/2
  flag_fuelcut/1 -> Not_cal/1(In1)
  Not_cal/1(Out1) -> Product2/1
  flag_IdleStop/1 -> Not_cal1/1(In1)
  Not_cal1/1(Out1) -> Product2/2
  Product1/1 -> trq_ENG_PNT_Nm/1  "trq_ENG_PNT_Nm"

== system METI_Thermal_ver01_Jmaab_2018b_Intg/Vehicle/ENG_PNT/ENG_Plant/Coldstart_Additional_friction_calc2 ==
  note: スロットル開度0の時の
      | 軸トルクを読み出し
  T_ENGOil_degC : Inport
  w_ENG_PNT_radps : Inport  Port=2
  1-D Lookup Table : Lookup_n-D  NumberOfTableDimensions=1  BreakpointsForDimension1=ENG_PNT_Cold_friction_gain_x_T_ENGOil  Table=ENG_PNT_Cold_friction_gain  InternalRulePriority=Speed  RndMeth=Simplest  InputSameDT=on
  2-D Lookup Table : Lookup_n-D  BreakpointsForDimension1=ENG_PNT_trq_Nm_map_y_throttle  BreakpointsForDimension2=ENG_PNT_trq_Nm_map_x_rpm  Table=ENG_PNT_trq_Nm_map  ExtrapMethod=Clip  UseLastTableValue=on  RndMeth=Simplest  InputSameDT=on
  Add : Sum  Inputs=+-
  Constant1 : Constant  Value=0
  Product : Product
  radpsec2rpm : Gain  Gain=radpsec2rpm
  Additional_friction : Outport
  wires:
  T_ENGOil_degC/1 -> 1-D Lookup Table/1
  w_ENG_PNT_radps/1 -> radpsec2rpm/1
  radpsec2rpm/1 -> 2-D Lookup Table/2
  Constant1/1 -> 2-D Lookup Table/1
  2-D Lookup Table/1 -> Add/2, Product/2
  1-D Lookup Table/1 -> Product/1
  Add/1 -> Additional_friction/1
  Product/1 -> Add/1

== system METI_Thermal_ver01_Jmaab_2018b_Intg/Vehicle/ENG_PNT/ENG_Plant/Coldstart_Heat_flux_gain_calc ==
  T_ENGOil_degC : Inport
  1-D Lookup Table : Lookup_n-D  NumberOfTableDimensions=1  BreakpointsForDimension1=ENG_PNT_Heatflux2ENGOil_gain_x_T_ENGOil  Table=ENG_PNT_Heatflux2ENGOil_gain  InternalRulePriority=Speed  RndMeth=Simplest  InputSameDT=on
  Heat_flux_gain : Outport
  wires:
  T_ENGOil_degC/1 -> 1-D Lookup Table/1
  1-D Lookup Table/1 -> Heat_flux_gain/1

== system METI_Thermal_ver01_Jmaab_2018b_Intg/Vehicle/ENG_PNT/ENG_Plant/Coldstart_Heat_flux_gain_calc1 ==
  T_ENG_Cylinder_Head_degC : Inport
  1-D Lookup Table : Lookup_n-D  NumberOfTableDimensions=1  BreakpointsForDimension1=ENG_PNT_Heatflux2Cylinder_Head_gain_x_T_Coolant  Table=ENG_PNT_Heatflux2Cylinder_Head_gain  InternalRulePriority=Speed  RndMeth=Simplest  InputSameDT=on
  Heat_flux_gain : Outport
  wires:
  T_ENG_Cylinder_Head_degC/1 -> 1-D Lookup Table/1
  1-D Lookup Table/1 -> Heat_flux_gain/1

== system METI_Thermal_ver01_Jmaab_2018b_Intg/Vehicle/ENG_PNT/ENG_Plant/K->degC1 ==
  K : Inport
  Constant2 : Constant  Value=K2degC
  Sum : Sum  Inputs=++|
  degC : Outport
  wires:
  K/1 -> Sum/2
  Constant2/1 -> Sum/1
  Sum/1 -> degC/1

== system METI_Thermal_ver01_Jmaab_2018b_Intg/Vehicle/ENG_PNT/ENG_Plant/K->degC6 ==
  K : Inport
  Constant2 : Constant  Value=K2degC
  Sum : Sum  Inputs=++|
  degC : Outport
  wires:
  K/1 -> Sum/2
  Constant2/1 -> Sum/1
  Sum/1 -> degC/1

== system METI_Thermal_ver01_Jmaab_2018b_Intg/Vehicle/PTTH/ATM_PNT/degC->K ==
  degC : Inport
  Constant2 : Constant  Value=degC2K
  Sum : Sum  Inputs=++|
  K : Outport
  wires:
  degC/1 -> Sum/2
  Constant2/1 -> Sum/1
  Sum/1 -> K/1

== system METI_Thermal_ver01_Jmaab_2018b_Intg/Vehicle/PTTH/ATM_PNT/degC->K1 ==
  degC : Inport
  Constant2 : Constant  Value=degC2K
  Sum : Sum  Inputs=++|
  K : Outport
  wires:
  Sum/1 -> K/1
  Constant2/1 -> Sum/1
  degC/1 -> Sum/2

== system METI_Thermal_ver01_Jmaab_2018b_Intg/Vehicle/PTTH/ATM_PNT/degC->K2 ==
  degC : Inport
  Constant2 : Constant  Value=degC2K
  Sum : Sum  Inputs=++|
  K : Outport
  wires:
  degC/1 -> Sum/2
  Constant2/1 -> Sum/1
  Sum/1 -> K/1

== system METI_Thermal_ver01_Jmaab_2018b_Intg/Vehicle/PTTH/ATM_PNT/degC->K3 ==
  degC : Inport
  Constant2 : Constant  Value=degC2K
  Sum : Sum  Inputs=++|
  K : Outport
  wires:
  Sum/1 -> K/1
  Constant2/1 -> Sum/1
  degC/1 -> Sum/2

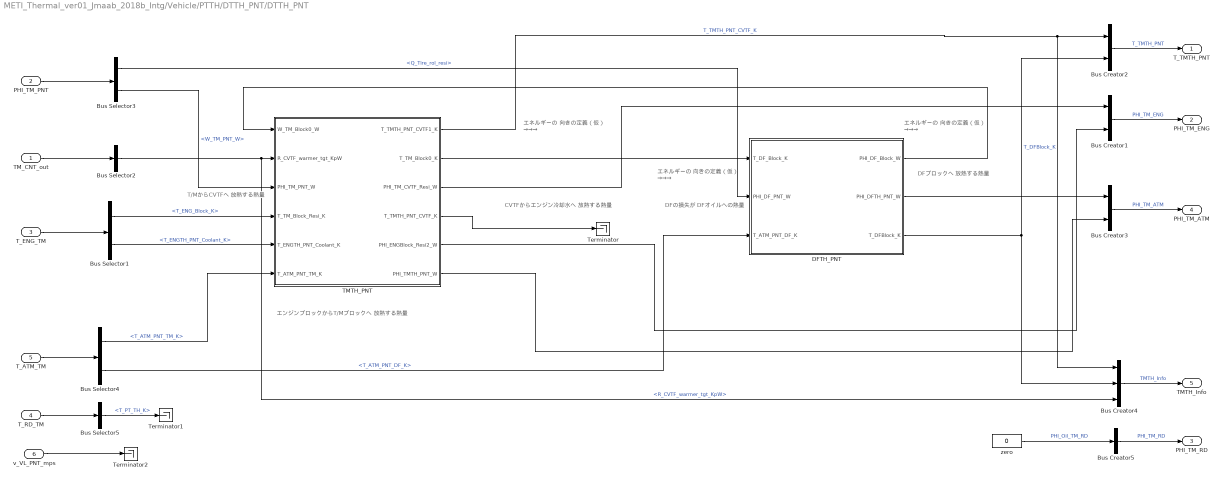
== system METI_Thermal_ver01_Jmaab_2018b_Intg/Vehicle/PTTH/DTTH_PNT/DTTH_PNT ==
  note: DFブロックへ
      | 放熱する熱量
  note: CVTFからエンジン冷却水へ
      | 放熱する熱量
  note: エンジンブロックからT/Mブロックへ
      | 放熱する熱量
  note: エネルギーの
      | 向きの定義（仮）
      | →→→
  note: エネルギーの
      | 向きの定義（仮）
      | →→→
  note: エネルギーの
      | 向きの定義（仮）
      | →→→
  note: T/MからCVTFへ
      | 放熱する熱量
  note: DFの損失が
      | DFオイルへの熱量
  TM_CNT_out : Inport
  PHI_TM_PNT : Inport  Port=2
  T_ENG_TM : Inport  Port=3
  T_RD_TM : Inport  Port=4
  T_ATM_TM : Inport  Port=5
  v_VL_PNT_mps : Inport  Port=6
  Bus Creator1 : BusCreator  Inputs=2
  Bus Creator2 : BusCreator  Inputs=2
  Bus Creator3 : BusCreator  Inputs=2
  Bus Creator4 : BusCreator  Inputs=3
  Bus Creator5 : BusCreator  Inputs=1
  Bus Selector1 : BusSelector  OutputSignals=T_ENG_Block_K,T_ENGTH_PNT_Coolant_K
  Bus Selector2 : BusSelector  OutputSignals=R_CVTF_warmer_tgt_KpW
  Bus Selector3 : BusSelector  OutputSignals=Q_Tire_rol_resi,W_TM_PNT_W
  Bus Selector4 : BusSelector  OutputSignals=T_ATM_PNT_TM_K,T_ATM_PNT_DF_K
  Bus Selector5 : BusSelector  OutputSignals=T_PT_TH_K
  DFTH_PNT : Subsystem
      mask Display: image(imread('picture\回転変換.png'))
  TMTH_PNT : Subsystem
      mask Display: image(imread('picture\image\トランスミッション02.jpg'))
  Terminator : Terminator
  Terminator1 : Terminator
  Terminator2 : Terminator
  zero : Constant  Value=0
  T_TMTH_PNT : Outport
  PHI_TM_ENG : Outport  Port=2
  PHI_TM_RD : Outport  Port=3
  PHI_TM_ATM : Outport  Port=4
  TMTH_Info : Outport  Port=5
  wires:
  DFTH_PNT/2(PHI_DFTH_PNT_W) -> Bus Creator3/1
  Bus Selector4/2 -> DFTH_PNT/3(T_ATM_PNT_DF_K)  "<T_ATM_PNT_DF_K>"
  TMTH_PNT/4(T_TMTH_PNT_CVTF_K) -> Terminator/1
  TMTH_PNT/2(T_TM_Block0_K) -> DFTH_PNT/1(T_DF_Block_K)
  DFTH_PNT/1(PHI_DF_Block_W) -> TMTH_PNT/1(W_TM_Block0_W)
  TMTH_PNT/6(PHI_TMTH_PNT_W) -> Bus Creator3/2
  TMTH_PNT/5(PHI_ENGBlock_Resi2_W) -> Bus Creator1/2
  TMTH_PNT/3(PHI_TM_CVTF_Resi_W) -> Bus Creator1/1
  T_ENG_TM/1 -> Bus Selector1/1
  Bus Selector1/1 -> TMTH_PNT/4(T_TM_Block_Resi_K)  "<T_ENG_Block_K>"
  Bus Selector1/2 -> TMTH_PNT/5(T_ENGTH_PNT_Coolant_K)  "<T_ENGTH_PNT_Coolant_K>"
  TMTH_PNT/1(T_TMTH_PNT_CVTF1_K) -> Bus Creator4/1, Bus Creator2/1  "T_TMTH_PNT_CVTF_K"
  DFTH_PNT/3(T_DFBlock_K) -> Bus Creator4/2, Bus Creator2/2  "T_DFBlock_K"
  Bus Creator2/1 -> T_TMTH_PNT/1  "T_TMTH_PNT"
  Bus Creator1/1 -> PHI_TM_ENG/1  "PHI_TM_ENG"
  Bus Creator3/1 -> PHI_TM_ATM/1  "PHI_TM_ATM"
  Bus Creator4/1 -> TMTH_Info/1  "TMTH_Info"
  PHI_TM_PNT/1 -> Bus Selector3/1
  Bus Selector3/2 -> TMTH_PNT/3(PHI_TM_PNT_W)  "<W_TM_PNT_W>"
  Bus Selector3/1 -> DFTH_PNT/2(PHI_DF_PNT_W)  "<Q_Tire_rol_resi>"
  TM_CNT_out/1 -> Bus Selector2/1
  Bus Selector2/1 -> Bus Creator4/3, TMTH_PNT/2(R_CVTF_warmer_tgt_KpW)  "<R_CVTF_warmer_tgt_KpW>"
  T_ATM_TM/1 -> Bus Selector4/1
  Bus Selector4/1 -> TMTH_PNT/6(T_ATM_PNT_TM_K)  "<T_ATM_PNT_TM_K>"
  Bus Creator5/1 -> PHI_TM_RD/1  "PHI_TM_RD"
  zero/1 -> Bus Creator5/1  "PHI_Oil_TM_RD"
  T_RD_TM/1 -> Bus Selector5/1
  Bus Selector5/1 -> Terminator1/1  "<T_PT_TH_K>"
  v_VL_PNT_mps/1 -> Terminator2/1

== system METI_Thermal_ver01_Jmaab_2018b_Intg/Vehicle/PTTH/ENGTH_PNT/ENGTH ==
  note: エンジンオイル
      | 熱容量
  note: エンジン冷却水
      | 熱容量
  note: エンジンブロック
      | 熱容量
  note: 冷却水からラジエターへ
      | 放熱する熱量
  note: エネルギーの
      | 向きの定義（仮）
      | →→→
  note: エンジン燃焼室からシリンダヘッドへ
      | 放熱する熱量
  note: エンジンからエンジンオイルへ
      | 放熱する熱量
  note: エネルギーの
      | 向きの定義（仮）
      | →→→
  note: エネルギーの
      | 向きの定義（仮）
      | →→→
  note: エネルギーの
      | 向きの定義（仮）
      | →→→
  note: エネルギーの
      | 向きの定義（仮）
      | →→→
  note: エネルギーの
      | 向きの定義（仮）
      | →→→
  note: エネルギーの
      | 向きの定義（仮）
      | →→→
  note: エンジンブロックからT/Mブロックへ
      | 放熱する熱量
  note: シリンダヘッド
      | 熱容量
  note: エネルギーの
      | 向きの定義（仮）
      | →→→
  V_ENG_CNT_WP_V : Inport
  PHI_ENGBlock_W : Inport  Port=2
  PHI_ENG_PNT_Head_W : Inport  Port=3
  PHI_ENG_PNT_Oil_W : Inport  Port=4
  T_ATM_PNT_ENG_K : Inport  Port=5
  PHI_TM_CVTF_Resi_W : Inport  Port=6
  PHI_ENGCoolant_W1 : Inport  Port=7
  Add : Sum
  Coolant_Heat_Capacity : Subsystem
  Cylinder_Head2Coolant_Heat_Resistance : Subsystem
  ENGBlock2Air_Heat_Resistance : Subsystem
  ENGBlock2Coolant_Heat_Resistance : Subsystem
  ENGBlock_Heat_Capacity : Subsystem
  ENGOil2Coolant_Heat_Resistance : Subsystem
  ENGOil_Heat_Capacity : Subsystem
  ENGOil_Heat_Capacity1 : Subsystem
  Water_Pump : Subsystem
  T_ENGTH_PNT_Coolant_K : Outport
  T_ENG_Block_K : Outport  Port=2
  T_ENGTH_PNT_Oil_K : Outport  Port=3
  T_ENGTH_PNT_Head_K : Outport  Port=4
  PHI_ENGTH_PNT_W : Outport  Port=5
  wires:
  PHI_TM_CVTF_Resi_W/1 -> Add/1
  Add/1 -> Coolant_Heat_Capacity/4(PHI_Coolant2_W)  "PHI_ENGCoolant_W"
  ENGOil_Heat_Capacity/1(T_ENGOil2_K) -> ENGOil2Coolant_Heat_Resistance/1(T_ENGOil_Resi2_K)
  ENGOil2Coolant_Heat_Resistance/2(PHI_Coolant_Resi3_W) -> Coolant_Heat_Capacity/3(PHI_Coolant3_W)
  PHI_ENGCoolant_W1/1 -> Add/2
  PHI_ENG_PNT_Head_W/1 -> ENGOil_Heat_Capacity1/1(PHI_Cylinder_Head1_W)
  ENGBlock_Heat_Capacity/3(T_ENGBlock1_K) -> ENGBlock2Coolant_Heat_Resistance/2(T_ENGBlock_Resi1_K)
  ENGBlock_Heat_Capacity/1(T_ENGBlock3_K) -> ENGBlock2Air_Heat_Resistance/1(T_ENGBlock_Resi3_K)
  ENGOil_Heat_Capacity1/1(T_Cylinder_Head1_K) -> T_ENGTH_PNT_Head_K/1  "T_Cylinder_Head0_K"
  Cylinder_Head2Coolant_Heat_Resistance/1(PHI_Coolant_Resi1_W) -> Coolant_Heat_Capacity/2(PHI_Coolant1_W)
  Cylinder_Head2Coolant_Heat_Resistance/2(PHI_Cylinder_Head_Resi2_W) -> ENGOil_Heat_Capacity1/2(PHI_Cylinder_Head2_W)
  Water_Pump/1(Qv_Coolant_m3ps) -> Cylinder_Head2Coolant_Heat_Resistance/2(Qv_Coolant_m3ps)
  ENGBlock_Heat_Capacity/2(T_ENGBlock2_K) -> T_ENG_Block_K/1  "T_ENG_Block_K"
  PHI_ENGBlock_W/1 -> ENGBlock_Heat_Capacity/3(PHI_ENGBlock2_W)
  V_ENG_CNT_WP_V/1 -> Water_Pump/1(ENG_PNT_Voltage_WP_V)
  ENGOil_Heat_Capacity1/2(T_Cylinder_Head2_K) -> Cylinder_Head2Coolant_Heat_Resistance/3(T_Cylinder_Head_Resi2_K)
  ENGBlock2Coolant_Heat_Resistance/1(PHI_Coolant_Resi4_W) -> Coolant_Heat_Capacity/1(PHI_Coolant4_W)
  Coolant_Heat_Capacity/4(T_Coolant3_K) -> ENGOil2Coolant_Heat_Resistance/2(T_Coolant_Resi3_K)
  ENGBlock2Air_Heat_Resistance/1(PHI_ENGBlock_Resi3_W) -> ENGBlock_Heat_Capacity/1(PHI_ENGBlock3_W)
  ENGOil2Coolant_Heat_Resistance/1(PHI_ENGOil_Resi2_W) -> ENGOil_Heat_Capacity/1(PHI_ENGOil2_W)
  Coolant_Heat_Capacity/2(T_Coolant4_K) -> ENGBlock2Coolant_Heat_Resistance/1(T_Coolant_Resi4_K)
  T_ATM_PNT_ENG_K/1 -> ENGBlock2Air_Heat_Resistance/2(T_ENG_Air_Resi1_K)
  ENGBlock2Coolant_Heat_Resistance/2(PHI_ENGBlock_Resi1_W) -> ENGBlock_Heat_Capacity/2(PHI_ENGBlock1_W)
  Coolant_Heat_Capacity/3(T_Coolant2_K) -> T_ENGTH_PNT_Coolant_K/1  "T_ENGTH_PNT_Coolant_K"
  Coolant_Heat_Capacity/1(T_Coolant1_K) -> Cylinder_Head2Coolant_Heat_Resistance/1(T_Coolant_Resi1_K)
  ENGBlock2Air_Heat_Resistance/2(PHI_ENG_Air_Resi1_W) -> PHI_ENGTH_PNT_W/1  "PHI_ENGTH_PNT_W"
  ENGOil_Heat_Capacity/2(T_ENGOil1_K) -> T_ENGTH_PNT_Oil_K/1  "T_ENGOil0_K"
  PHI_ENG_PNT_Oil_W/1 -> ENGOil_Heat_Capacity/2(PHI_ENGOil1_W)

== system METI_Thermal_ver01_Jmaab_2018b_Intg/Vehicle/PTTH/RDTH_PNT/RDTH ==
  note: サーモスタット
  note: エネルギーの
      | 向きの定義（仮）
      | →→→
  note: エネルギーの
      | 向きの定義（仮）
      | →→→
  RD_PNT_Voltage_RDFan_V : Inport
  v_VL_PNT_kmph : Inport  Port=2
  T_ENGTH_PNT_Coolant_K : Inport  Port=3
  T_ATM_PNT_RD_K : Inport  Port=4
  ENGBlock2Coolant_Heat_Resistance : Subsystem
  RDCoolant2Air_Heat_Resistance : Subsystem
  RDCoolant_Heat_Capacity : Subsystem
  RD_Core_Heat_Resi_Calc : Subsystem
  T_RDCoolant_degC : Outport
  PHI_RDTH_PNT_W : Outport  Port=2
  PHI_RD_Air_Resi_W : Outport  Port=3
  tag scope: RD_PNT_RDCore_Heat_Resi_KpW=global
  wires:
  T_ATM_PNT_RD_K/1 -> RDCoolant2Air_Heat_Resistance/1(T_RD_Air_Resi_K)
  RDCoolant_Heat_Capacity/2(T_RDCoolant2_K) -> T_RDCoolant_degC/1, RDCoolant2Air_Heat_Resistance/3(T_RDCoolant_Resi2_K)  "T_RDCoolant_degC"
  RDCoolant_Heat_Capacity/1(T_RDCoolant1_K) -> ENGBlock2Coolant_Heat_Resistance/1(T_RDCoolant_Resi1_K)
  RD_Core_Heat_Resi_Calc/1("RD_PNT_RDCore_Heat_Resi_KpW ") -> [RD_PNT_RDCore_Heat_Resi_KpW], RDCoolant2Air_Heat_Resistance/2("RD_PNT_RDCore_Heat_Resi_KpW ")
  RDCoolant2Air_Heat_Resistance/1(PHI_RD_Air_Resi1_W) -> PHI_RD_Air_Resi_W/1  "PHI_RD_Air_Resi_W"
  T_ENGTH_PNT_Coolant_K/1 -> ENGBlock2Coolant_Heat_Resistance/2(T_Thermostat_Resi1_K)
  ENGBlock2Coolant_Heat_Resistance/2(PHI_Thermostat_Resi1_W) -> PHI_RDTH_PNT_W/1  "PHI_RDTH_PNT_W"
  RDCoolant2Air_Heat_Resistance/2(PHI_RDCoolant_Resi2_W) -> RDCoolant_Heat_Capacity/2(PHI_RDCoolant2_W)
  ENGBlock2Coolant_Heat_Resistance/1(PHI_RDCoolant_Resi1_W) -> RDCoolant_Heat_Capacity/1(PHI_RDCoolant1_W)
  RD_PNT_Voltage_RDFan_V/1 -> RD_Core_Heat_Resi_Calc/1(RD_PNT_Voltage_RDFan_V)
  v_VL_PNT_kmph/1 -> RD_Core_Heat_Resi_Calc/2(v_VL_PNT_kmph)
